simulink model "prob3bias"  (R2019a)
settings: Solver=VariableStepAuto  StartTime=0.0  StopTime=10.0  RelTol=1e-3
values from neighbouring files (symbols this model uses):
  accBias = 1E-3 * g    [prob3main.m]
  C1 = 3/tau    [prob3main.m]
  C2 = 2*schuler^2 + 3/tau/tau    [prob3main.m]
  C3 = 1/(tau^3)    [prob3main.m]
  schuler = sqrt(g/R)    [prob3main.m]
undefined symbols (not defined in the file or in its folder): altBias
settings Model: Creator=hyunwoong  LastModifiedBy=hyunwoong

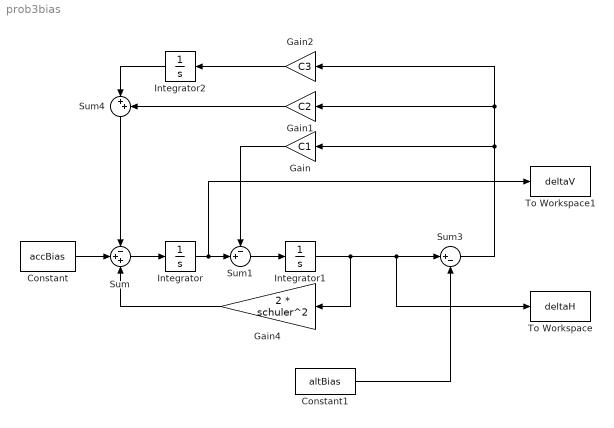
== system prob3bias ==
  Constant : Constant  Value=accBias
  Constant1 : Constant  Value=altBias
  Gain : Gain  Gain=C1
  Gain1 : Gain  Gain=C2
  Gain2 : Gain  Gain=C3
  Gain4 : Gain  Gain=2 * schuler^2
  Integrator : Integrator
  Integrator1 : Integrator
  Integrator2 : Integrator
  Sum : Sum  Inputs=-++
  Sum1 : Sum  Inputs=-+|
  Sum3 : Sum  Inputs=|+-
  Sum4 : Sum  Inputs=|++
  To Workspace : ToWorkspace  VariableName=deltaH  SaveFormat=Timeseries  SampleTime=-1
  To Workspace1 : ToWorkspace  VariableName=deltaV  SaveFormat=Timeseries  SampleTime=-1
  wires:
  Constant/1 -> Sum/2
  Sum/1 -> Integrator/1
  Integrator/1 -> To Workspace1/1, Sum1/2
  Sum1/1 -> Integrator1/1
  Gain/1 -> Sum1/1
  Gain2/1 -> Integrator2/1
  Gain1/1 -> Sum4/2
  Integrator2/1 -> Sum4/1
  Sum4/1 -> Sum/1
  Sum3/1 -> Gain1/1, Gain2/1, Gain/1
  Integrator1/1 -> To Workspace/1, Sum3/1, Gain4/1
  Gain4/1 -> Sum/3
  Constant1/1 -> Sum3/2
